simulink model "coloumb_counting"  (R2023b)
settings: Solver=FixedStepAuto  StartTime=0.0  StopTime=3600  FixedStep=0.01  RelTol=1e-3
libraries: BatteryEstimators x9
settings Model: Creator=Mahdi  LastModifiedBy=Mahdi
settings OptimizationCC: DefaultParameterBehavior=Inlined  OptimizeBlockIOStorage=off  BufferReuse=off  ReuseModelBlockBuffer=off  GlobalBufferReuse=off  ExpressionFolding=off  EnableMemcpy=off  PassReuseOutputArgsAs=Individual arguments  LocalBlockOutputs=off  ZeroExternalMemoryAtStartup=off  ZeroInternalMemoryAtStartup=off  OptimizeDataStoreBuffers=off  BusAssignmentInplaceUpdate=off  OptimizationLevel=level0  OptimizationCustomize=off  EfficientTunableParamExpr=on
settings DebuggingCC: ParameterTunabilityLossMsg=error
settings HardwareCC: ProdBitPerInt=16  ProdBitPerPointer=16  ProdBitPerSizeT=16  ProdBitPerPtrDiffT=16  ProdLargestAtomicFloat=None  ProdWordSize=16  ProdHWDeviceType=STMicroelectronics->ST10/Super10
settings SFSimCC: MATLABDynamicMemAlloc=off
settings RTWCC: Description=Embedded Coder  SystemTargetFile=ert.tlc  TemplateMakefile=ert_default_tmf  BuildConfiguration=Debug
settings CodeAppCC: ForceParamTrailComments=on  IgnoreCustomStorageClasses=off  OperatorAnnotations=on  SimulinkDataObjDesc=on  SFDataObjDesc=on  InsertBlockDesc=on
settings ERTTargetCC: TargetLangStandard=C99 (ISO)  GenerateSampleERTMain=on  InlinedParameterPlacement=NonHierarchical  ERTCustomFileTemplate=example_file_process.tlc

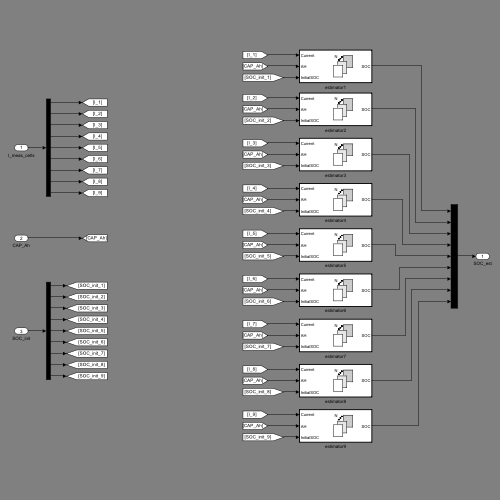
[thumbnail: Simulink's stored preview of the top-level diagram]
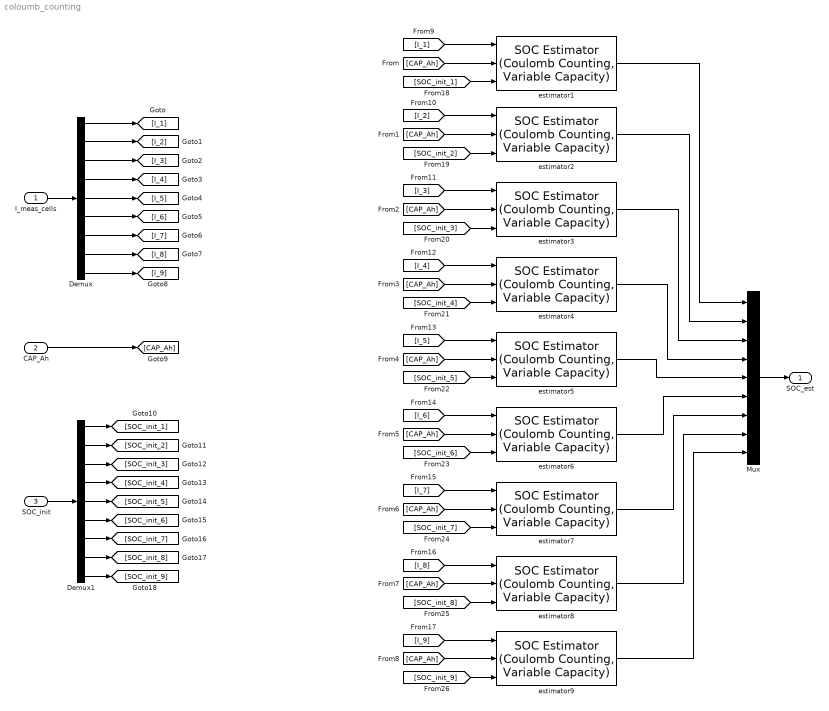
== system coloumb_counting ==
  I_meas_cells : Inport
  CAP_Ah : Inport  Port=2
  SOC_init : Inport  Port=3
  Demux : Demux  Outputs=9
  Demux1 : Demux  Outputs=9
  Mux : Mux  Inputs=9
  estimator{1..9} (9 alike) : BatteryEstimators/SOC Estimator (Coulomb Counting, Variable Capacity)  CurrentInputPartition=on  Ts=-1
      settings: LibrarySourceBlock=|
      | batt_sl_lib/Estimators/SOC Estimator
      | (Coulomb Counting, Variable Capacity)
  SOC_est : Outport
  wires:
  I_meas_cells/1 -> Demux/1
  Demux/1 -> [I_1]
  Demux/2 -> [I_2]
  Demux/3 -> [I_3]
  Demux/4 -> [I_4]
  Demux/5 -> [I_5]
  Demux/6 -> [I_6]
  Demux/7 -> [I_7]
  Demux/8 -> [I_8]
  Demux/9 -> [I_9]
  CAP_Ah/1 -> [CAP_Ah]
  [CAP_Ah] -> estimator1/2
  [CAP_Ah] -> estimator2/2
  [CAP_Ah] -> estimator3/2
  [CAP_Ah] -> estimator4/2
  [CAP_Ah] -> estimator5/2
  [CAP_Ah] -> estimator6/2
  [CAP_Ah] -> estimator7/2
  [CAP_Ah] -> estimator8/2
  [CAP_Ah] -> estimator9/2
  Demux1/4 -> [SOC_init_4]
  Demux1/5 -> [SOC_init_5]
  Demux1/6 -> [SOC_init_6]
  Demux1/1 -> [SOC_init_1]
  Demux1/8 -> [SOC_init_8]
  Demux1/3 -> [SOC_init_3]
  Demux1/7 -> [SOC_init_7]
  SOC_init/1 -> Demux1/1
  Demux1/9 -> [SOC_init_9]
  Demux1/2 -> [SOC_init_2]
  [I_1] -> estimator1/1
  [SOC_init_1] -> estimator1/3
  [I_2] -> estimator2/1
  [SOC_init_2] -> estimator2/3
  [I_3] -> estimator3/1
  [SOC_init_3] -> estimator3/3
  [I_4] -> estimator4/1
  [SOC_init_4] -> estimator4/3
  [I_5] -> estimator5/1
  [SOC_init_5] -> estimator5/3
  [I_6] -> estimator6/1
  [SOC_init_6] -> estimator6/3
  [I_7] -> estimator7/1
  [SOC_init_7] -> estimator7/3
  [I_8] -> estimator8/1
  [SOC_init_8] -> estimator8/3
  [I_9] -> estimator9/1
  [SOC_init_9] -> estimator9/3
  estimator1/1 -> Mux/1
  estimator2/1 -> Mux/2
  estimator3/1 -> Mux/3
  estimator4/1 -> Mux/4
  estimator5/1 -> Mux/5
  estimator6/1 -> Mux/6
  estimator7/1 -> Mux/7
  estimator8/1 -> Mux/8
  estimator9/1 -> Mux/9
  Mux/1 -> SOC_est/1
